simulink model "E040R1_D1_remap_add_iqcot_20260629"  (R2024b)
settings: Solver=VariableStepAuto  StartTime=0.0  StopTime=0.52e-3  MaxStep=5e-9  RelTol=1e-3
undefined symbols (not defined in the file): A_init, A_lower, A_upper, Cout, DCR_L1, DCR_L2, DCR_L3, DCR_L4, E040_Calibration_Enable, E040_Current_Deadband, E040_Current_Limit_A, E040_Dwell_Time, E040_Fallback_K_T, E040_I_Add_High, E040_IL_Sense_Gain1, E040_IL_Sense_Gain2, E040_IL_Sense_Gain3, E040_IL_Sense_Gain4, E040_K_T, E040_LoadStep_Time, E040_Min_Scale, E040_New_Phase_Ramp_Time, E040_New_Phase_Ton_Limit_Frac, E040_Order_Relock_Window, E040_Post_Add_Recovery_Band, E040_Post_Add_Reentry_Delay, E040_Post_Add_Ton_Recovery_Enable, E040_Post_Add_Ton_Recovery_Max, E040_Post_Add_Ton_Recovery_Window, E040_Sense_Confidence, E040_Severe_Overshoot_Band, E040_T_Trim_Max, E040_TonDiff_Enable, E040_V_Error_Budget, E040_V_Error_Hard_Limit, E040_Variant_Mode, E040_Vref, ESR_C, IdealIQCOT_Enable, IL_adc_counts_per_A, IL_pk_limit_adc_neg, IL_pk_limit_adc_pos, Iload_final, Iload_initial, Iph, Iqcot_enable, kappa_cmd, Kiqcot, Kvc_iqcot, L, Lambda0_iqcot, Lambda_m2, rho_cmd, Ri_iqcot, t_load_step, Tblank, Tdead, Tiqcot_leak, Toff_min, Ton_cmd ... (+11)
libraries: simulink x29, spsCurrentMeasurementLib x8, spsMosfetLib x8, spsSeriesRLCBranchLib x5, spsVoltageMeasurementLib x5, spsDCVoltageSourceLib x4, spsControlledCurrentSourceLib x1, spsGroundLib x1, spspowerguiLib x1
(part 2 of 2)

== system E040R1_D1_remap_add_iqcot_20260629/GateDriver_1Phase2/OnDelay1 ==
  u : Inport
  Compare To Constant : simulink/Logic and Bit Operations/Compare To Constant  relop=>=  const=Tdead  OutDataTypeStr=boolean
  Data Type Conversion : DataTypeConversion  OutDataTypeStr=double  SaturateOnIntegerOverflow=off  RndMeth=Floor
  Integrator : Integrator  ExternalReset=level
  Logical Operator : Logic  Operator=NOT  AllPortsSameDT=off  OutDataTypeStr=boolean
  y : Outport
  wires:
  u/1 -> Data Type Conversion/1, Logical Operator/1
  Logical Operator/1 -> Integrator/2
  Data Type Conversion/1 -> Integrator/1
  Integrator/1 -> Compare To Constant/1
  Compare To Constant/1 -> y/1

== system E040R1_D1_remap_add_iqcot_20260629/GateDriver_1Phase3/OnDelay ==
  u : Inport
  Compare To Constant : simulink/Logic and Bit Operations/Compare To Constant  relop=>=  const=Tdead  OutDataTypeStr=boolean
  Data Type Conversion : DataTypeConversion  OutDataTypeStr=double  SaturateOnIntegerOverflow=off  RndMeth=Floor
  Integrator : Integrator  ExternalReset=level
  Logical Operator : Logic  Operator=NOT  AllPortsSameDT=off  OutDataTypeStr=boolean
  y : Outport
  wires:
  u/1 -> Data Type Conversion/1, Logical Operator/1
  Logical Operator/1 -> Integrator/2
  Data Type Conversion/1 -> Integrator/1
  Integrator/1 -> Compare To Constant/1
  Compare To Constant/1 -> y/1

== system E040R1_D1_remap_add_iqcot_20260629/GateDriver_1Phase3/OnDelay1 ==
  u : Inport
  Compare To Constant : simulink/Logic and Bit Operations/Compare To Constant  relop=>=  const=Tdead  OutDataTypeStr=boolean
  Data Type Conversion : DataTypeConversion  OutDataTypeStr=double  SaturateOnIntegerOverflow=off  RndMeth=Floor
  Integrator : Integrator  ExternalReset=level
  Logical Operator : Logic  Operator=NOT  AllPortsSameDT=off  OutDataTypeStr=boolean
  y : Outport
  wires:
  u/1 -> Data Type Conversion/1, Logical Operator/1
  Logical Operator/1 -> Integrator/2
  Data Type Conversion/1 -> Integrator/1
  Integrator/1 -> Compare To Constant/1
  Compare To Constant/1 -> y/1

== system E040R1_D1_remap_add_iqcot_20260629/GateDriver_1Phase4/OnDelay ==
  u : Inport
  Compare To Constant : simulink/Logic and Bit Operations/Compare To Constant  relop=>=  const=Tdead  OutDataTypeStr=boolean
  Data Type Conversion : DataTypeConversion  OutDataTypeStr=double  SaturateOnIntegerOverflow=off  RndMeth=Floor
  Integrator : Integrator  ExternalReset=level
  Logical Operator : Logic  Operator=NOT  AllPortsSameDT=off  OutDataTypeStr=boolean
  y : Outport
  wires:
  u/1 -> Data Type Conversion/1, Logical Operator/1
  Logical Operator/1 -> Integrator/2
  Data Type Conversion/1 -> Integrator/1
  Integrator/1 -> Compare To Constant/1
  Compare To Constant/1 -> y/1

== system E040R1_D1_remap_add_iqcot_20260629/GateDriver_1Phase4/OnDelay1 ==
  u : Inport
  Compare To Constant : simulink/Logic and Bit Operations/Compare To Constant  relop=>=  const=Tdead  OutDataTypeStr=boolean
  Data Type Conversion : DataTypeConversion  OutDataTypeStr=double  SaturateOnIntegerOverflow=off  RndMeth=Floor
  Integrator : Integrator  ExternalReset=level
  Logical Operator : Logic  Operator=NOT  AllPortsSameDT=off  OutDataTypeStr=boolean
  y : Outport
  wires:
  u/1 -> Data Type Conversion/1, Logical Operator/1
  Logical Operator/1 -> Integrator/2
  Data Type Conversion/1 -> Integrator/1
  Integrator/1 -> Compare To Constant/1
  Compare To Constant/1 -> y/1

== matlab function E040R1_D1_remap_add_iqcot_20260629/Ideal_Digital_IQCOT_Request/IQCOT_Event_Core ==
  data: e_v input double size=1; REQ_iqcot output double size=1; IL1 input double size=1; IL2 input double size=1; IL3 input double size=1; IL4 input double size=1; phase_idx input double size=1; tr_reset input double size=1; enable input double size=1; Ts_ctrl_in input double size=1; Lambda0_in input double size=1; Lambda_m2_in input double size=1; rho_cmd_in input double size=1; Ri_in input double size=1; Kvc_in input double size=1; Vc_bias_in input double size=1; kappa_cmd_in input double size=1; A_init_in input double size=1; A_lower_in input double size=1; A_upper_in input double size=1; A_iqcot output double size=1; Lambda_i output double size=1; h_iqcot output double size=1; IL_sel output double size=1; vc_ctrl output double size=1
function [REQ_iqcot,A_iqcot,Lambda_i,h_iqcot,IL_sel,vc_ctrl] = IQCOT_Event_Core(e_v,IL1,IL2,IL3,IL4,phase_idx,tr_reset,enable,Ts_ctrl_in,Lambda0_in,Lambda_m2_in,rho_cmd_in,Ri_in,Kvc_in,Vc_bias_in,kappa_cmd_in,A_init_in,A_lower_in,A_upper_in)
%#codegen
REQ_iqcot = 0.0;
A_iqcot = 0.0;
Lambda_i = 0.0;
h_iqcot = 0.0;
IL_sel = 0.0;
vc_ctrl = 0.0;
persistent Astate reset_prev phase_prev
if isempty(Astate)
    Astate = double(A_init_in);
end
if isempty(reset_prev)
    reset_prev = 0.0;
end
if isempty(phase_prev)
    phase_prev = 0.0;
end
p = floor(double(phase_idx));
p = mod(p, 4);
if p == 0
    IL_sel = IL1;
elseif p == 1
    IL_sel = IL2;
elseif p == 2
    IL_sel = IL3;
else
    IL_sel = IL4;
end
Ri_eff = Ri_in * exp(kappa_cmd_in);
vc_ctrl = Vc_bias_in + Kvc_in * e_v;
h_iqcot = vc_ctrl - Ri_eff * IL_sel;
Lambda_i = Lambda0_in * (1 + rho_cmd_in) + Lambda_m2_in * cos(pi * p);
if Lambda_i < eps
    Lambda_i = eps;
end
A_update = Astate + Ts_ctrl_in * h_iqcot;
if A_update < A_lower_in
    A_update = A_lower_in;
end
if A_update > A_upper_in
    A_update = A_upper_in;
end
REQ_iqcot = double((enable > 0.5) && (A_update >= Lambda_i));
A_iqcot = A_update;
reset_rise = (tr_reset > 0.5) && (reset_prev <= 0.5);
phase_change = (p ~= phase_prev);
if enable <= 0.5
    Astate = A_init_in;
elseif reset_rise || phase_change
    Astate = A_init_in;
else
    Astate = A_update;
end
reset_prev = double(tr_reset);
phase_prev = p;

== matlab function E040R1_D1_remap_add_iqcot_20260629/E040_TonActual1 ==
  data: qh input boolean; Ton_actual output double; t input double
function Ton_actual = ton_actual_estimator(qh, t)
%#codegen
persistent q_prev t_rise last_width
if isempty(q_prev)
    q_prev = 0.0;
end
if isempty(t_rise)
    t_rise = 0.0;
end
if isempty(last_width)
    last_width = 0.0;
end
is_high = double(qh > 0.5);
if is_high > 0.5 && q_prev <= 0.5
    t_rise = t;
elseif is_high <= 0.5 && q_prev > 0.5
    last_width = max(0.0, t - t_rise);
end
Ton_actual = last_width;
q_prev = is_high;

== matlab function E040R1_D1_remap_add_iqcot_20260629/E040_TonActual2 ==
  data: qh input boolean; Ton_actual output double; t input double
function Ton_actual = ton_actual_estimator(qh, t)
%#codegen
persistent q_prev t_rise last_width
if isempty(q_prev)
    q_prev = 0.0;
end
if isempty(t_rise)
    t_rise = 0.0;
end
if isempty(last_width)
    last_width = 0.0;
end
is_high = double(qh > 0.5);
if is_high > 0.5 && q_prev <= 0.5
    t_rise = t;
elseif is_high <= 0.5 && q_prev > 0.5
    last_width = max(0.0, t - t_rise);
end
Ton_actual = last_width;
q_prev = is_high;

== matlab function E040R1_D1_remap_add_iqcot_20260629/E040_TonActual3 ==
  data: qh input boolean; Ton_actual output double; t input double
function Ton_actual = ton_actual_estimator(qh, t)
%#codegen
persistent q_prev t_rise last_width
if isempty(q_prev)
    q_prev = 0.0;
end
if isempty(t_rise)
    t_rise = 0.0;
end
if isempty(last_width)
    last_width = 0.0;
end
is_high = double(qh > 0.5);
if is_high > 0.5 && q_prev <= 0.5
    t_rise = t;
elseif is_high <= 0.5 && q_prev > 0.5
    last_width = max(0.0, t - t_rise);
end
Ton_actual = last_width;
q_prev = is_high;

== matlab function E040R1_D1_remap_add_iqcot_20260629/E040_TonActual4 ==
  data: qh input boolean; Ton_actual output double; t input double
function Ton_actual = ton_actual_estimator(qh, t)
%#codegen
persistent q_prev t_rise last_width
if isempty(q_prev)
    q_prev = 0.0;
end
if isempty(t_rise)
    t_rise = 0.0;
end
if isempty(last_width)
    last_width = 0.0;
end
is_high = double(qh > 0.5);
if is_high > 0.5 && q_prev <= 0.5
    t_rise = t;
elseif is_high <= 0.5 && q_prev > 0.5
    last_width = max(0.0, t - t_rise);
end
Ton_actual = last_width;
q_prev = is_high;

== matlab function E040R1_D1_remap_add_iqcot_20260629/E040_A_ActivePhaseSupervisor ==
  data: req1 input boolean; req1o output boolean; req2 input boolean; req3 input boolean; req4 input boolean; ton1 input double; ton2 input double; ton3 input double; ton4 input double; il1 input double; il2 input double; il3 input double; il4 input double; vout input double; iload input double; t input double; t_step input double; variant_mode input double; I_add_high input double; dwell_time input double; new_phase_ramp_time input double; Vref input double; severe_overshoot_band input double; current_limit_A input double; TonDiff_enable input double; K_T input double; fallback_K_T input double; T_trim_Max input double; current_deadband input double; sense_confidence input double; calibration_enable input double; Verr_budget input double; Verr_hard input double; min_scale input double; new_phase_Ton_limit_frac input double; order_relock_window input double; post_add_reentry_delay input double; post_add_Ton_recovery_enable input double; post_add_Ton_recovery_max input double; post_add_Ton_recovery_window input double; post_add_recovery_band input double; req2o output boolean; req3o output boolean; req4o output boolean; ton1o output double; ton2o output double; ton3o output double; ton4o output double; active_phase_set output double; N_active output double; phase_add_request output double; phase_add_accept output double; phase_add_reject output double; phase_shed_request output double; phase_shed_accept output double; new_phase_ramp_state output double; residual_current_i output double; dwell_timer output double; protect_state output double; reentry_state output double; balance_recovery_state output double; sense_confidence_o output double; calibration_enable_o output double; a_S_mode output double; fallback_count_o output double; guard_clamp_count_o output double; trim1 output double; trim2 output double; trim3 output double; trim4 output double; REQ_accept1 output boolean; REQ_accept2 output boolean; REQ_accept3 output boolean; REQ_accept4 output boolean; REQ_reject_reason output double; logical_slot output double; physical_phase_selected output double; phase_add_reject_reason output double; new_phase_current_target output double; new_phase_Ton_limit output double; order_relock_state output double; order_relock_window_done output double; phase_order_error_rate_window output double; a_S_enable_after_add output double; current_limit_hit output double; post_add_Ton_recovery_active output double; post_add_Ton_recovery_usage output double
function [req1o,req2o,req3o,req4o,ton1o,ton2o,ton3o,ton4o,active_phase_set,N_active,phase_add_request,phase_add_accept,phase_add_reject,phase_shed_request,phase_shed_accept,new_phase_ramp_state,residual_current_i,dwell_timer,protect_state,reentry_state,balance_recovery_state,sense_confidence_o,calibration_enable_o,a_S_mode,fallback_count_o,guard_clamp_count_o,trim1,trim2,trim3,trim4,REQ_accept1,REQ_accept2,REQ_accept3,REQ_accept4,REQ_reject_reason,logical_slot,physical_phase_selected,phase_add_reject_reason,new_phase_current_target,new_phase_Ton_limit,order_relock_state,order_relock_window_done,phase_order_error_rate_window,a_S_enable_after_add,current_limit_hit,post_add_Ton_recovery_active,post_add_Ton_recovery_usage] = e040_supervisor(req1,req2,req3,req4,ton1,ton2,ton3,ton4,il1,il2,il3,il4,vout,iload,t,t_step,variant_mode,I_add_high,dwell_time,new_phase_ramp_time,Vref,severe_overshoot_band,current_limit_A,TonDiff_enable,K_T,fallback_K_T,T_trim_Max,current_deadband,sense_confidence,calibration_enable,Verr_budget,Verr_hard,min_scale,new_phase_Ton_limit_frac,order_relock_window,post_add_reentry_delay,post_add_Ton_recovery_enable,post_add_Ton_recovery_max,post_add_Ton_recovery_window,post_add_recovery_band)
%#codegen
req = [req1, req2, req3, req4] > 0.5;
tons = [ton1, ton2, ton3, ton4];
ils = [il1, il2, il3, il4];
base_ton = max(max(tons), 1.0e-12);
new_phase_Ton_limit = max(new_phase_Ton_limit_frac, 0.0) * base_ton;
if new_phase_Ton_limit <= 0.0
    new_phase_Ton_limit = base_ton;
end
new_phase_current_target = max(iload, 0.0) / 4.0;
phase_shed_request = 0.0;
phase_shed_accept = 0.0;
protect_state = 0.0;
phase_add_request = double((variant_mode > 0.5) && (iload > I_add_high));
if phase_add_request > 0.5
    dwell_timer = max(0.0, t - t_step);
else
    dwell_timer = 0.0;
end
overshoot_ok = vout <= (Vref + severe_overshoot_band);
current_limit_hit = double((current_limit_A > 0.0) && (max(abs(ils)) >= current_limit_A));
current_ok = current_limit_hit < 0.5;
dwell_ok = dwell_timer >= dwell_time;
if variant_mode < 0.5
    allow_add = false;
    add_time = t_step;
elseif variant_mode < 1.5
    allow_add = phase_add_request > 0.5;
    add_time = t_step;
else
    allow_add = (phase_add_request > 0.5) && overshoot_ok && current_ok && dwell_ok;
    add_time = t_step + dwell_time;
end
phase_add_accept = double(allow_add);
phase_add_reject = double((phase_add_request > 0.5) && ~allow_add);
phase_add_reject_reason = 0.0;
if phase_add_reject > 0.5
    if ~dwell_ok
        phase_add_reject_reason = 2.0;
    elseif ~overshoot_ok
        phase_add_reject_reason = 3.0;
    elseif ~current_ok
        phase_add_reject_reason = 4.0;
    else
        phase_add_reject_reason = 1.0;
    end
end
if phase_add_accept > 0.5 && new_phase_ramp_time > 0.0
    ramp = min(max((t - add_time) / new_phase_ramp_time, 0.0), 1.0);
elseif phase_add_accept > 0.5
    ramp = 1.0;
else
    ramp = 0.0;
end
new_phase_ramp_state = ramp;
ramp_done = (phase_add_accept > 0.5) && (ramp >= 0.999);
order_relock_done = (phase_add_accept > 0.5) && (t >= add_time + max(new_phase_ramp_time, 0.0) + max(order_relock_window, 0.0));
order_relock_window_done = double(order_relock_done);
reentry_done = order_relock_done && (t >= add_time + max(new_phase_ramp_time, 0.0) + max(order_relock_window, 0.0) + max(post_add_reentry_delay, 0.0));
if phase_add_request < 0.5
    order_relock_state = 0.0;
elseif phase_add_accept < 0.5
    order_relock_state = 1.0;
elseif ~ramp_done
    order_relock_state = 2.0;
elseif ~order_relock_done
    order_relock_state = 3.0;
elseif ~reentry_done
    order_relock_state = 4.0;
else
    order_relock_state = 5.0;
end
if phase_add_accept > 0.5
    active_phase_set = [1.0, 1.0, 1.0, 1.0];
    N_active = 4.0;
    req_out = req;
    if req(1)
        logical_slot = 1.0; physical_phase_selected = 1.0;
    elseif req(2)
        logical_slot = 2.0; physical_phase_selected = 2.0;
    elseif req(3)
        logical_slot = 3.0; physical_phase_selected = 3.0;
    elseif req(4)
        logical_slot = 4.0; physical_phase_selected = 4.0;
    else
        logical_slot = 0.0; physical_phase_selected = 0.0;
    end
    ton_base = [ton1, min(ton2, new_phase_Ton_limit) * ramp, ton3, min(ton4, new_phase_Ton_limit) * ramp];
else
    active_phase_set = [1.0, 0.0, 1.0, 0.0];
    N_active = 2.0;
    req_out = [req(1) || req(3), false, req(2) || req(4), false];
    if req(1) || req(3)
        logical_slot = 1.0; physical_phase_selected = 1.0;
    elseif req(2) || req(4)
        logical_slot = 2.0; physical_phase_selected = 3.0;
    else
        logical_slot = 0.0; physical_phase_selected = 0.0;
    end
    ton_base = [ton1, 0.0, ton3, 0.0];
end
REQ_reject_reason = 0.0;
if any(req) && ~any(req_out)
    REQ_reject_reason = 1.0;
end
phase_order_error_rate_window = 0.0;
reentry_state = double(reentry_done);
a_S_enable_after_add = double((variant_mode >= 2.5) && (TonDiff_enable > 0.5) && reentry_done);
balance_enable = a_S_enable_after_add > 0.5;
a_S_mode = 0.0;
fallback_flag = 0.0;
guard_clamp = 0.0;
trim = [0.0, 0.0, 0.0, 0.0];
if balance_enable
    active_mask = active_phase_set > 0.5;
    low_confidence = (variant_mode >= 2.5) && (sense_confidence < 0.5);
    K_eff = K_T;
    if low_confidence
        K_eff = fallback_K_T;
        fallback_flag = 1.0;
        a_S_mode = 1.0;
    elseif calibration_enable > 0.5
        a_S_mode = 2.0;
    else
        K_eff = fallback_K_T;
        fallback_flag = 1.0;
        a_S_mode = 1.0;
    end
    denom = max(sum(double(active_mask)), 1.0);
    avg_i = sum(ils .* double(active_mask)) / denom;
    err = (ils - avg_i) .* double(active_mask);
    raw = -K_eff .* err;
    if max(abs(err)) < current_deadband
        raw = [0.0, 0.0, 0.0, 0.0];
    end
    trim = min(max(raw, -T_trim_Max), T_trim_Max);
    trim_mean = sum(trim .* double(active_mask)) / denom;
    trim = (trim - trim_mean) .* double(active_mask);
    max_trim = max(abs(trim));
    if T_trim_Max <= 0.0
        trim = [0.0, 0.0, 0.0, 0.0];
    elseif max_trim > T_trim_Max
        trim = trim .* (T_trim_Max / max_trim);
        guard_clamp = 1.0;
    end
    ev = abs(vout - Vref);
    denom_v = max(Verr_hard - Verr_budget, 1.0e-9);
    voltage_scale = 1.0 - max(ev - Verr_budget, 0.0) / denom_v;
    voltage_scale = min(max(voltage_scale, min_scale), 1.0);
    if voltage_scale < 0.999
        guard_clamp = 1.0;
    end
    trim = voltage_scale .* trim;
end
post_add_Ton_recovery_active = 0.0;
post_add_Ton_recovery_usage = 0.0;
recovery_boost = [0.0, 0.0, 0.0, 0.0];
recovery_deadline = add_time + max(new_phase_ramp_time, 0.0) + max(order_relock_window, 0.0) + max(post_add_Ton_recovery_window, 0.0);
recovery_ok = (post_add_Ton_recovery_enable > 0.5) && order_relock_done && (t <= recovery_deadline) && (vout < Vref - post_add_recovery_band) && current_ok;
if recovery_ok
    boost_cap = max(post_add_Ton_recovery_max - base_ton, 0.0);
    boost = min(0.10 * base_ton, boost_cap);
    active_mask = double(active_phase_set > 0.5);
    recovery_boost = boost .* active_mask;
    post_add_Ton_recovery_active = double(boost > 0.0);
    post_add_Ton_recovery_usage = boost / max(boost_cap, 1.0e-12);
end
ton_out = max([0.0, 0.0, 0.0, 0.0], ton_base + trim + recovery_boost);
req1o = req_out(1); req2o = req_out(2); req3o = req_out(3); req4o = req_out(4);
ton1o = ton_out(1); ton2o = ton_out(2); ton3o = ton_out(3); ton4o = ton_out(4);
residual_current_i = ils .* (1.0 - active_phase_set);
balance_recovery_state = double(balance_enable);
sense_confidence_o = sense_confidence;
calibration_enable_o = calibration_enable;
fallback_count_o = fallback_flag;
guard_clamp_count_o = guard_clamp;
trim1 = trim(1); trim2 = trim(2); trim3 = trim(3); trim4 = trim(4);
REQ_accept1 = req_out(1); REQ_accept2 = req_out(2); REQ_accept3 = req_out(3); REQ_accept4 = req_out(4);
